simulink model "exp7sim0x5B10x5D0x5B10x5D"  (R2024a)
settings: Solver=ode1  StartTime=0.0  StopTime=0.08  FixedStep=25e-6  RelTol=1e-3
libraries: spsIGBTDiodeLib x18, spsSeriesRLCBranchLib x6, spsDCVoltageSourceLib x3, spsGroundLib x3, spsThreePhaseSeriesRLCLoadLib x3, spsThreePhaseVIMeasurementLib x3, simulink x1, sps_lib x1
settings Model: Creator=archi  LastModifiedBy=kumar
settings RTWCC: GPUComputeCapability=3.5

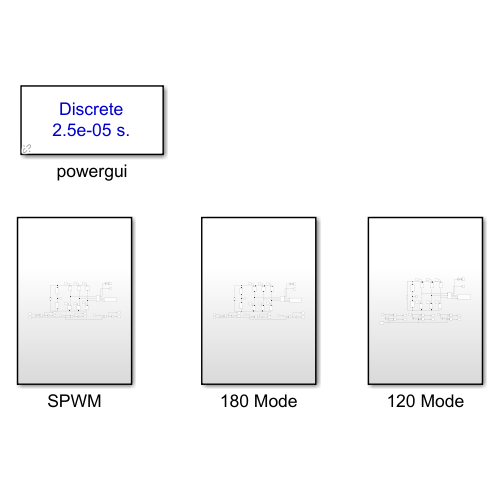
[thumbnail: Simulink's stored preview of the top-level diagram]
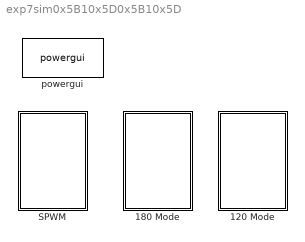
== system exp7sim0x5B10x5D0x5B10x5D ==
  120 Mode : Subsystem
  180 Mode : Subsystem
  SPWM : Subsystem
  powergui : sps_lib/powergui  Priority=1  SimulationMode=Discrete  SampleTime=25e-06  frequency=60  Iterations=50  frequencyindice=0  Pbase=100e6  ErrMax=1e-4  UnitsV=kV  UnitsW=MW  buscounter=0  FunctionMessages=off  echomessages=off  EnableUseOfTLC=off  CurrentSourceSwitches=off  DisableSnubberDevices=off  DisableRonSwitches=off  DisableVfSwitches=off  DisplayEquations=off  AutomaticDiscreteSolvers=off  SolverType=Tustin/Backward Euler (TBE)  Interpol=off  ExternalGateDelay=off  methode=off  Ts=100  x0status=blocks  SPID=on  SwTol=0  HookPort=off  NonlinearTolerance=1e-4  nMaxIteration=100  ContinueOnMaxIteration=off  RestoreLinks=warning  ResistiveCurrentMeasurement=off  Frange=[0:2:500]  Ylog=off  Xlog=on  ShowGrid=off  save=off  variable=ZData  structure=0  ZoomFFT=off  StartTime=0.0  cycles=1  DisplayStyle=1  fundamental=60  FreqAxis=off  MaxFrequency=1000  frequencyindicesteady=1  RmsSteady=1  display=off

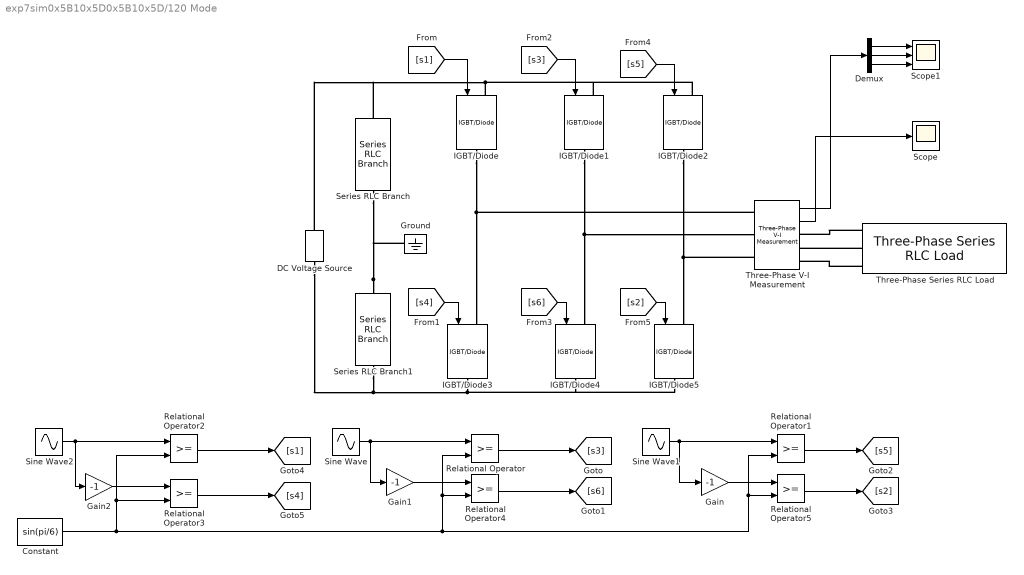
== system exp7sim0x5B10x5D0x5B10x5D/120 Mode ==
  Constant : Constant  Value=sin(pi/6)
  DC Voltage Source : spsDCVoltageSourceLib/DC Voltage Source  Amplitude=580  Measurements=None
  Demux : Demux  Outputs=3
  Gain : Gain  Gain=-1
  Gain1 : Gain  Gain=-1
  Gain2 : Gain  Gain=-1
  Ground : spsGroundLib/Ground  LConnTagsString=a
  IGBT/Diode{,1..5} (6 alike) : spsIGBTDiodeLib/IGBT//Diode  Ron=1e-3  Rs=1e5  Cs=inf  Measurements=off
  Relational Operator{,1..5} (6 alike) : RelationalOperator  OutDataTypeStr=boolean  RndMeth=Simplest  InputSameDT=off
  Scope : Scope
  Scope1 : Scope  NumInputPorts=3
  Series RLC Branch : spsSeriesRLCBranchLib/Series RLC Branch  LConnTagsString=__new0  RConnTagsString=__new0  BranchType=RC  Resistance=1  Inductance=1e-3  SetiL0=off  InitialCurrent=0  Capacitance=2200e-6  Setx0=off  InitialVoltage=0  Measurements=None
  Series RLC Branch1 : spsSeriesRLCBranchLib/Series RLC Branch  LConnTagsString=__new0  RConnTagsString=__new0  BranchType=RC  Resistance=1  Inductance=1e-3  SetiL0=off  InitialCurrent=0  Capacitance=2200e-6  Setx0=off  InitialVoltage=0  Measurements=None
  Sine Wave : Sin  Frequency=2*pi*50  Phase=2*pi/3  SampleTime=0
  Sine Wave1 : Sin  Frequency=2*pi*50  Phase=-2*pi/3  SampleTime=0
  Sine Wave2 : Sin  Frequency=2*pi*50  SampleTime=0
  Three-Phase Series RLC Load : spsThreePhaseSeriesRLCLoadLib/Three-Phase Series RLC Load  LConnTagsString=A|B|C  Configuration=Delta  NominalVoltage=230  Vabc=[1e3 1e3 1e3]  Vabcp=[1e3 1e3 1e3]  NominalFrequency=50  UnbalancedPower=off  ActivePower=1e3  InductivePower=0  CapacitivePower=0  Pabc=[10e3 9e3 11e3]  QLabc=[100 90 110]  QCabc=[100 90 110]  Pabcp=[10e3 9e3 11e3]  QLabcp=[100 90 110]  QCabcp=[100 90 110]  Measurements=None  LoadType=constant Z
  Three-Phase V-I Measurement : spsThreePhaseVIMeasurementLib/Three-Phase V-I Measurement  VoltageMeasurement=phase-to-ground  SetLabelV=off  LabelV=Vabc  Vpu=off  VpuLL=off  CurrentMeasurement=yes  SetLabelI=off  LabelI=Iabc  Ipu=off  Pbase=100e6  Vbase=500e3  OutputType=Complex  PhasorSimulation=off  PSBequivalent=0
  wires:
  Constant/1 -> Relational Operator5/2, Relational Operator1/2, Relational Operator4/2, Relational Operator/2, Relational Operator3/2, Relational Operator2/2
  Relational Operator/1 -> [s3]
  [s5] -> IGBT/Diode2/1
  [s6] -> IGBT/Diode4/1
  Relational Operator1/1 -> [s5]
  Relational Operator2/1 -> [s1]
  [s1] -> IGBT/Diode/1
  [s3] -> IGBT/Diode1/1
  Sine Wave1/1 -> Gain/1, Relational Operator1/1
  Sine Wave2/1 -> Gain2/1, Relational Operator2/1
  [s4] -> IGBT/Diode3/1
  Sine Wave/1 -> Gain1/1, Relational Operator/1
  [s2] -> IGBT/Diode5/1
  Relational Operator4/1 -> [s6]
  Relational Operator3/1 -> [s4]
  Gain1/1 -> Relational Operator4/1
  Gain/1 -> Relational Operator5/1
  Relational Operator5/1 -> [s2]
  Gain2/1 -> Relational Operator3/1
  Three-Phase V-I Measurement/1 -> Demux/1
  Demux/2 -> Scope1/2
  Demux/1 -> Scope1/1
  Demux/3 -> Scope1/3
  Three-Phase V-I Measurement/2 -> Scope/1
  connections:
  DC Voltage Source/LConn1 -- Series RLC Branch1/RConn1 -- IGBT/Diode3/RConn1 -- IGBT/Diode5/RConn1 -- IGBT/Diode4/RConn1
  IGBT/Diode2/RConn1 -- Three-Phase V-I Measurement/LConn3 -- IGBT/Diode5/LConn1
  IGBT/Diode2/LConn1 -- IGBT/Diode1/LConn1 -- Series RLC Branch/LConn1 -- DC Voltage Source/RConn1 -- IGBT/Diode/LConn1
  IGBT/Diode/RConn1 -- Three-Phase V-I Measurement/LConn1 -- IGBT/Diode3/LConn1
  IGBT/Diode1/RConn1 -- Three-Phase V-I Measurement/LConn2 -- IGBT/Diode4/LConn1
  Three-Phase Series RLC Load/LConn3 -- Three-Phase V-I Measurement/RConn3
  Three-Phase Series RLC Load/LConn2 -- Three-Phase V-I Measurement/RConn2
  Three-Phase Series RLC Load/LConn1 -- Three-Phase V-I Measurement/RConn1
  Series RLC Branch1/LConn1 -- Series RLC Branch/RConn1 -- Ground/LConn1

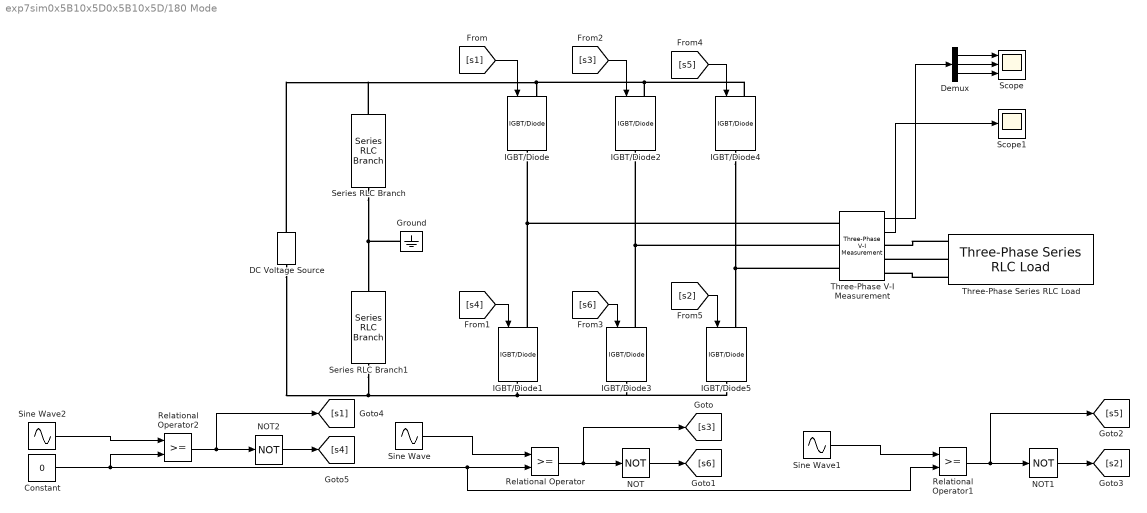
== system exp7sim0x5B10x5D0x5B10x5D/180 Mode ==
  Constant : Constant  Value=0
  DC Voltage Source : spsDCVoltageSourceLib/DC Voltage Source  Amplitude=580  Measurements=None
  Demux : Demux  Outputs=3
  Ground : spsGroundLib/Ground  LConnTagsString=a
  IGBT/Diode{,1..5} (6 alike) : spsIGBTDiodeLib/IGBT//Diode  Ron=1e-3  Rs=1e5  Cs=inf  Measurements=off
  NOT : Logic  Operator=NOT  IconShape=distinctive  AllPortsSameDT=off  OutDataTypeStr=boolean
  NOT1 : Logic  Operator=NOT  IconShape=distinctive  AllPortsSameDT=off  OutDataTypeStr=boolean
  NOT2 : Logic  Operator=NOT  IconShape=distinctive  AllPortsSameDT=off  OutDataTypeStr=boolean
  Relational Operator : RelationalOperator  OutDataTypeStr=boolean  RndMeth=Simplest  InputSameDT=off
  Relational Operator1 : RelationalOperator  OutDataTypeStr=boolean  RndMeth=Simplest  InputSameDT=off
  Relational Operator2 : RelationalOperator  OutDataTypeStr=boolean  RndMeth=Simplest  InputSameDT=off
  Scope : Scope  NumInputPorts=3
  Scope1 : Scope
  Series RLC Branch : spsSeriesRLCBranchLib/Series RLC Branch  LConnTagsString=__new0  RConnTagsString=__new0  BranchType=RC  Resistance=1  Inductance=1e-3  SetiL0=off  InitialCurrent=0  Capacitance=2200e-6  Setx0=off  InitialVoltage=0  Measurements=None
  Series RLC Branch1 : spsSeriesRLCBranchLib/Series RLC Branch  LConnTagsString=__new0  RConnTagsString=__new0  BranchType=RC  Resistance=1  Inductance=1e-3  SetiL0=off  InitialCurrent=0  Capacitance=2200e-6  Setx0=off  InitialVoltage=0  Measurements=None
  Sine Wave : Sin  Amplitude=0.8  Frequency=314  Phase=2*pi/3  SampleTime=0
  Sine Wave1 : Sin  Amplitude=0.8  Frequency=314  Phase=-2*pi/3  SampleTime=0
  Sine Wave2 : Sin  Amplitude=0.8  Frequency=314  SampleTime=0
  Three-Phase Series RLC Load : spsThreePhaseSeriesRLCLoadLib/Three-Phase Series RLC Load  LConnTagsString=A|B|C  Configuration=Delta  NominalVoltage=230  Vabc=[1e3 1e3 1e3]  Vabcp=[1e3 1e3 1e3]  NominalFrequency=50  UnbalancedPower=off  ActivePower=1e3  InductivePower=400  CapacitivePower=0  Pabc=[10e3 9e3 11e3]  QLabc=[100 90 110]  QCabc=[100 90 110]  Pabcp=[10e3 9e3 11e3]  QLabcp=[100 90 110]  QCabcp=[100 90 110]  Measurements=None  LoadType=constant Z
  Three-Phase V-I Measurement : spsThreePhaseVIMeasurementLib/Three-Phase V-I Measurement  VoltageMeasurement=phase-to-ground  SetLabelV=off  LabelV=Vabc  Vpu=off  VpuLL=off  CurrentMeasurement=yes  SetLabelI=off  LabelI=Iabc  Ipu=off  Pbase=100e6  Vbase=500e3  OutputType=Complex  PhasorSimulation=off  PSBequivalent=0
  wires:
  Demux/3 -> Scope/3
  Constant/1 -> Relational Operator2/2, Relational Operator1/2, Relational Operator/2
  Relational Operator/1 -> [s3], NOT/1
  [s5] -> IGBT/Diode4/1
  Demux/2 -> Scope/2
  NOT/1 -> [s6]
  [s6] -> IGBT/Diode3/1
  Relational Operator1/1 -> [s5], NOT1/1
  Relational Operator2/1 -> [s1], NOT2/1
  NOT2/1 -> [s4]
  [s1] -> IGBT/Diode/1
  [s3] -> IGBT/Diode2/1
  Three-Phase V-I Measurement/2 -> Scope1/1
  NOT1/1 -> [s2]
  Sine Wave1/1 -> Relational Operator1/1
  Sine Wave2/1 -> Relational Operator2/1
  Three-Phase V-I Measurement/1 -> Demux/1
  [s4] -> IGBT/Diode1/1
  Sine Wave/1 -> Relational Operator/1
  [s2] -> IGBT/Diode5/1
  Demux/1 -> Scope/1
  connections:
  Series RLC Branch1/RConn1 -- DC Voltage Source/LConn1 -- IGBT/Diode1/RConn1 -- IGBT/Diode5/RConn1 -- IGBT/Diode3/RConn1
  IGBT/Diode4/RConn1 -- Three-Phase V-I Measurement/LConn3 -- IGBT/Diode5/LConn1
  IGBT/Diode1/LConn1 -- Three-Phase V-I Measurement/LConn1 -- IGBT/Diode/RConn1
  IGBT/Diode3/LConn1 -- Three-Phase V-I Measurement/LConn2 -- IGBT/Diode2/RConn1
  IGBT/Diode2/LConn1 -- Series RLC Branch/LConn1 -- DC Voltage Source/RConn1 -- IGBT/Diode/LConn1 -- IGBT/Diode4/LConn1
  Three-Phase Series RLC Load/LConn2 -- Three-Phase V-I Measurement/RConn2
  Series RLC Branch/RConn1 -- Ground/LConn1 -- Series RLC Branch1/LConn1
  Three-Phase Series RLC Load/LConn1 -- Three-Phase V-I Measurement/RConn1
  Three-Phase Series RLC Load/LConn3 -- Three-Phase V-I Measurement/RConn3

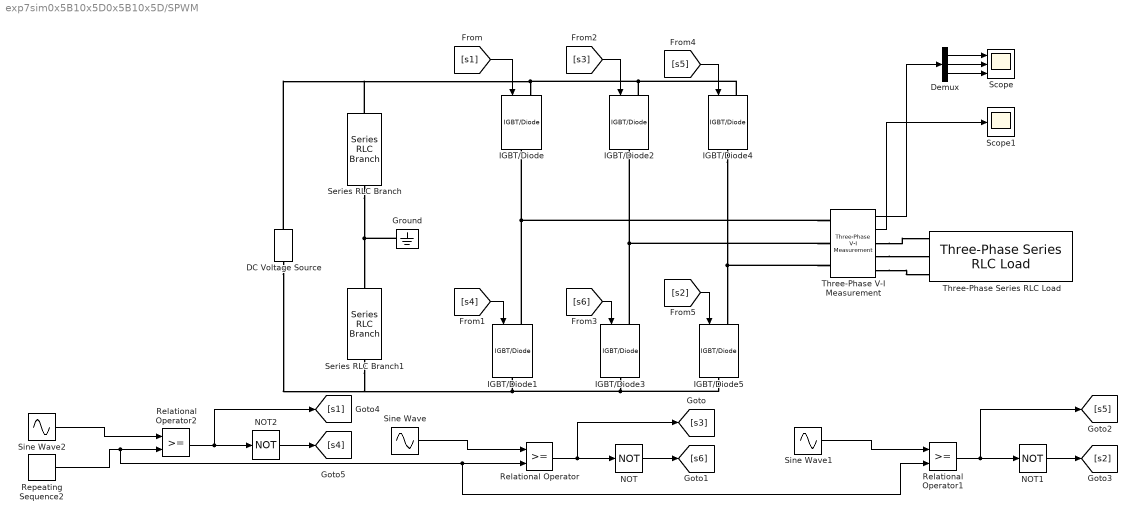
== system exp7sim0x5B10x5D0x5B10x5D/SPWM ==
  DC Voltage Source : spsDCVoltageSourceLib/DC Voltage Source  Amplitude=580  Measurements=None
  Demux : Demux  Outputs=3
  Ground : spsGroundLib/Ground  LConnTagsString=a
  IGBT/Diode{,1..5} (6 alike) : spsIGBTDiodeLib/IGBT//Diode  Ron=1e-3  Rs=1e5  Cs=inf  Measurements=off
  NOT : Logic  Operator=NOT  IconShape=distinctive  AllPortsSameDT=off  OutDataTypeStr=boolean
  NOT1 : Logic  Operator=NOT  IconShape=distinctive  AllPortsSameDT=off  OutDataTypeStr=boolean
  NOT2 : Logic  Operator=NOT  IconShape=distinctive  AllPortsSameDT=off  OutDataTypeStr=boolean
  Relational Operator : RelationalOperator  OutDataTypeStr=boolean  RndMeth=Simplest  InputSameDT=off
  Relational Operator1 : RelationalOperator  OutDataTypeStr=boolean  RndMeth=Simplest  InputSameDT=off
  Relational Operator2 : RelationalOperator  OutDataTypeStr=boolean  RndMeth=Simplest  InputSameDT=off
  Repeating Sequence2 : simulink/Sources/Repeating Sequence  rep_seq_t=[0 1 2 3 4]/4000  rep_seq_y=[0 1 0 -1 0]
  Scope : Scope  NumInputPorts=3
  Scope1 : Scope
  Series RLC Branch : spsSeriesRLCBranchLib/Series RLC Branch  LConnTagsString=__new0  RConnTagsString=__new0  BranchType=RC  Resistance=1  Inductance=1e-3  SetiL0=off  InitialCurrent=0  Capacitance=2200e-6  Setx0=off  InitialVoltage=0  Measurements=None
  Series RLC Branch1 : spsSeriesRLCBranchLib/Series RLC Branch  LConnTagsString=__new0  RConnTagsString=__new0  BranchType=RC  Resistance=1  Inductance=1e-3  SetiL0=off  InitialCurrent=0  Capacitance=2200e-6  Setx0=off  InitialVoltage=0  Measurements=None
  Sine Wave : Sin  Amplitude=0.8  Frequency=314  Phase=2*pi/3  SampleTime=0
  Sine Wave1 : Sin  Amplitude=0.8  Frequency=314  Phase=-2*pi/3  SampleTime=0
  Sine Wave2 : Sin  Amplitude=0.8  Frequency=314  SampleTime=0
  Three-Phase Series RLC Load : spsThreePhaseSeriesRLCLoadLib/Three-Phase Series RLC Load  LConnTagsString=A|B|C  Configuration=Delta  NominalVoltage=230  Vabc=[1e3 1e3 1e3]  Vabcp=[1e3 1e3 1e3]  NominalFrequency=50  UnbalancedPower=off  ActivePower=1e3  InductivePower=400  CapacitivePower=0  Pabc=[10e3 9e3 11e3]  QLabc=[100 90 110]  QCabc=[100 90 110]  Pabcp=[10e3 9e3 11e3]  QLabcp=[100 90 110]  QCabcp=[100 90 110]  Measurements=None  LoadType=constant Z
  Three-Phase V-I Measurement : spsThreePhaseVIMeasurementLib/Three-Phase V-I Measurement  VoltageMeasurement=phase-to-ground  SetLabelV=off  LabelV=Vabc  Vpu=off  VpuLL=off  CurrentMeasurement=yes  SetLabelI=off  LabelI=Iabc  Ipu=off  Pbase=100e6  Vbase=500e3  OutputType=Complex  PhasorSimulation=off  PSBequivalent=0
  wires:
  Demux/3 -> Scope/3
  Repeating Sequence2/1 -> Relational Operator1/2, Relational Operator/2, Relational Operator2/2
  Relational Operator/1 -> [s3], NOT/1
  [s5] -> IGBT/Diode4/1
  Demux/2 -> Scope/2
  NOT/1 -> [s6]
  [s6] -> IGBT/Diode3/1
  Relational Operator1/1 -> [s5], NOT1/1
  Relational Operator2/1 -> [s1], NOT2/1
  NOT2/1 -> [s4]
  [s1] -> IGBT/Diode/1
  [s3] -> IGBT/Diode2/1
  Three-Phase V-I Measurement/2 -> Scope1/1
  NOT1/1 -> [s2]
  Sine Wave1/1 -> Relational Operator1/1
  Sine Wave2/1 -> Relational Operator2/1
  Three-Phase V-I Measurement/1 -> Demux/1
  [s4] -> IGBT/Diode1/1
  Sine Wave/1 -> Relational Operator/1
  [s2] -> IGBT/Diode5/1
  Demux/1 -> Scope/1
  connections:
  IGBT/Diode3/RConn1 -- Series RLC Branch1/RConn1 -- DC Voltage Source/LConn1 -- IGBT/Diode1/RConn1 -- IGBT/Diode5/RConn1
  IGBT/Diode4/RConn1 -- Three-Phase V-I Measurement/LConn3 -- IGBT/Diode5/LConn1
  IGBT/Diode1/LConn1 -- Three-Phase V-I Measurement/LConn1 -- IGBT/Diode/RConn1
  IGBT/Diode3/LConn1 -- Three-Phase V-I Measurement/LConn2 -- IGBT/Diode2/RConn1
  IGBT/Diode2/LConn1 -- Series RLC Branch/LConn1 -- DC Voltage Source/RConn1 -- IGBT/Diode/LConn1 -- IGBT/Diode4/LConn1
  Three-Phase V-I Measurement/RConn2 -- Three-Phase Series RLC Load/LConn2
  Series RLC Branch/RConn1 -- Ground/LConn1 -- Series RLC Branch1/LConn1
  Three-Phase V-I Measurement/RConn1 -- Three-Phase Series RLC Load/LConn1
  Three-Phase V-I Measurement/RConn3 -- Three-Phase Series RLC Load/LConn3
